simulink model "idle_speed_control"  (R2017b)
settings: Solver=VariableStepAuto  StartTime=0.0  StopTime=10.0  RelTol=1e-3
undefined symbols (not defined in the file): a, aL, ap, b, bL, bp, G, k, n0, phi
settings Model: Creator=ernst  LastModifiedBy=ernst

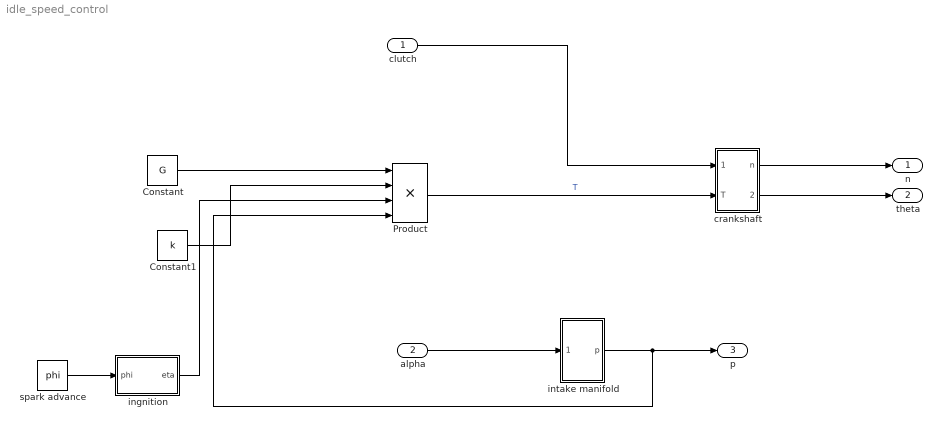
== system idle_speed_control ==
  clutch : Inport
  alpha : Inport  Port=2
  Constant : Constant  Value=G
  Constant1 : Constant  Value=k
  Product : Product  Inputs=4
  crankshaft : Subsystem
  ingnition : Subsystem
  intake manifold : Subsystem
  spark advance : Constant  Value=phi
  n : Outport
  theta : Outport  Port=2
  p : Outport  Port=3
  wires:
  spark advance/1 -> ingnition/1(phi)
  alpha/1 -> intake manifold/1(alpha)
  intake manifold/1(p) -> Product/4, p/1
  clutch/1 -> crankshaft/1(clutch)
  crankshaft/1(n) -> n/1
  crankshaft/2(theta) -> theta/1
  Constant1/1 -> Product/2
  Constant/1 -> Product/1
  ingnition/1(eta) -> Product/3
  Product/1 -> crankshaft/2(T)  "T"

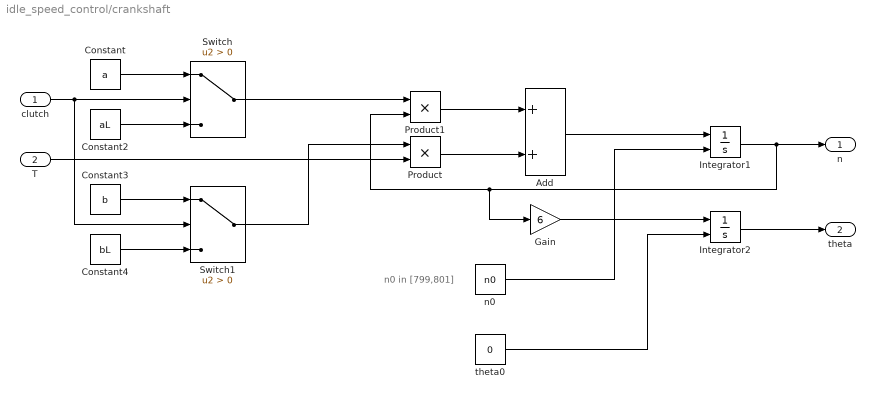
== system idle_speed_control/crankshaft ==
  note: n0 in [799,801]
  clutch : Inport
  T : Inport  Port=2
  Add : Sum
  Constant : Constant  Value=a
  Constant2 : Constant  Value=aL
  Constant3 : Constant  Value=b
  Constant4 : Constant  Value=bL
  Gain : Gain  Gain=6
  Integrator1 : Integrator  InitialConditionSource=external
  Integrator2 : Integrator  InitialConditionSource=external
  Product : Product
  Product1 : Product
  Switch : Switch  Criteria=u2 > Threshold
  Switch1 : Switch  Criteria=u2 > Threshold
  n0 : Constant  Value=n0
  theta0 : Constant  Value=0
  n : Outport
  theta : Outport  Port=2
  wires:
  Constant3/1 -> Switch1/1
  Product1/1 -> Add/1
  Add/1 -> Integrator1/1
  Product/1 -> Add/2
  theta0/1 -> Integrator2/2
  Constant/1 -> Switch/1
  Switch/1 -> Product1/1
  Constant4/1 -> Switch1/3
  Switch1/1 -> Product/1
  Gain/1 -> Integrator2/1
  clutch/1 -> Switch1/2, Switch/2
  T/1 -> Product/2
  n0/1 -> Integrator1/2
  Integrator2/1 -> theta/1
  Constant2/1 -> Switch/3
  Integrator1/1 -> n/1, Product1/2, Gain/1

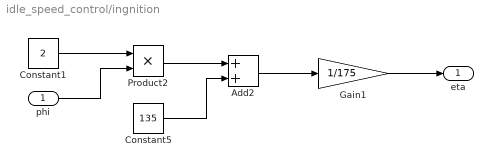
== system idle_speed_control/ingnition ==
  phi : Inport
  Add2 : Sum
  Constant1 : Constant  Value=2
  Constant5 : Constant  Value=135
  Gain1 : Gain  Gain=1/175
  Product2 : Product
  eta : Outport
  wires:
  Constant5/1 -> Add2/2
  phi/1 -> Product2/2
  Constant1/1 -> Product2/1
  Product2/1 -> Add2/1
  Gain1/1 -> eta/1
  Add2/1 -> Gain1/1

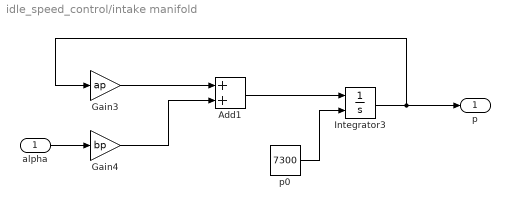
== system idle_speed_control/intake manifold ==
  alpha : Inport
  Add1 : Sum
  Gain3 : Gain  Gain=ap
  Gain4 : Gain  Gain=bp
  Integrator3 : Integrator  InitialConditionSource=external
  p0 : Constant  Value=7300
  p : Outport
  wires:
  Add1/1 -> Integrator3/1
  Gain4/1 -> Add1/2
  Gain3/1 -> Add1/1
  alpha/1 -> Gain4/1
  p0/1 -> Integrator3/2
  Integrator3/1 -> p/1, Gain3/1
